simulink model "PDControllerModifiedToWork"  (R2020b)
settings: Solver=VariableStepAuto  StartTime=0.0  StopTime=30  RelTol=1e-3
values from neighbouring files (symbols this model uses):
  Arm = dhfunc(descriptor,d,a,alpha,theta,m,I,r,G,Jm,fv)    [Test.m]    (also in TestZone.m = dhfunc(descriptor,d,a,alpha,theta,m,I,r,G,Jm, Fv); TestZone2.m = dhfunc(descriptor,d,a,alpha,theta,m,I,r,G,Jm, Fc, Fv); TestZone2WithSingularity.m = dhfunc(descriptor,d,a,alpha,theta,m,I,r,G,Jm, Fv); dhfunc.m = SerialLink(LinkList, 'name', 'Arm'))
  Kd = eye(6)*kd    [TestZone.m]    (also in TestZone2.m = eye(3)*kd; TestZone2WithSingularity.m; Workspace.mat = [1 0 0 0 0 0 0 1 0 0 0 0 ... (36 elements, 6x6)])
  Kp = eye(6)*kp    [TestZone.m]    (also in TestZone2.m = eye(3)*kp; TestZone2WithSingularity.m; Workspace.mat = [1 0 0 0 0 0 0 1 0 0 0 0 ... (36 elements, 6x6)])
  Od = [1 0 0 1; 0 1 0 2; 0 0 1 3; 0 0 0 1]    [TestZone.m]    (also in Workspace.mat = [0.764842187284 0.644217687238 0 0 -0.644217687238 0.7648421)
  qdintial = [0,0,0,0,0,0]    [TestZone.m]    (also in Workspace.mat = [0 0 0])
  qintial = [0,0,0,0,0,0]    [TestZone.m]    (also in Workspace.mat = [0 0 0])
libraries: roblocks x1
settings Model: Creator=William Weiss  LastModifiedBy=kylej

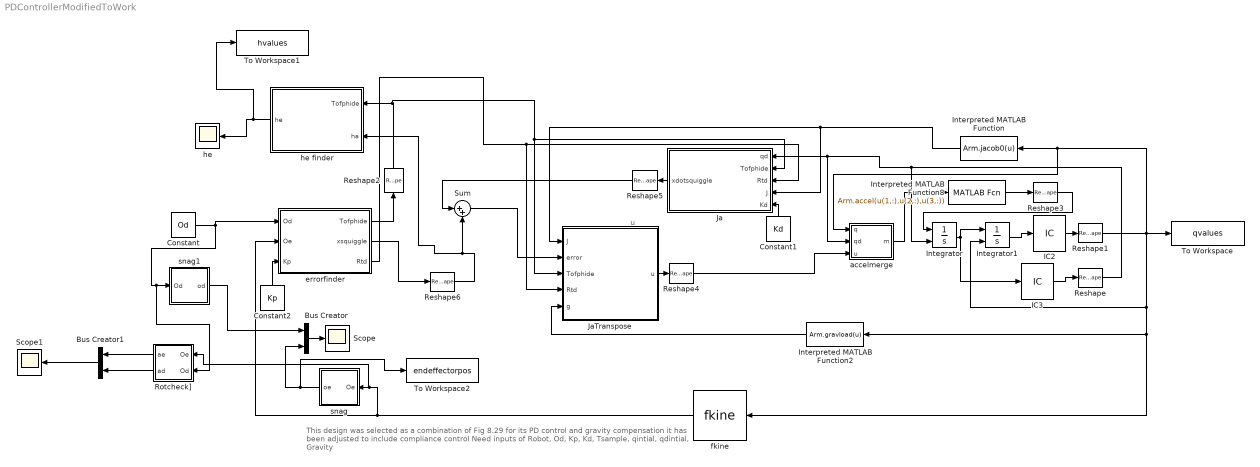
== system PDControllerModifiedToWork ==
  note: This design was selected as a combination of Fig 8.29 for its PD control and gravity compensation
      | it has been adjusted to include compliance control
      |
      | Need inputs of Robot, Od, Kp, Kd, Tsample, qintial, qdintial, Gravity
  note: u
  Bus Creator : BusCreator  Inputs=2
  Bus Creator1 : BusCreator  Inputs=2
  Constant : Constant  Value=Od
  Constant1 : Constant  Value=Kd
  Constant2 : Constant  Value=Kp
  IC2 : InitialCondition  Value=qintial
  IC3 : InitialCondition  Value=qdintial
  Integrator : Integrator  InitialConditionSource=external  ZeroCross=off
  Integrator1 : Integrator  InitialConditionSource=external  ZeroCross=off
  Interpreted MATLAB Function : MATLABFcn  MATLABFcn=Arm.jacob0(u)  Output1D=off
  Interpreted MATLAB Function2 : MATLABFcn  MATLABFcn=Arm.gravload(u)  Output1D=off
  Interpreted MATLAB Function8 : MATLABFcn  MATLABFcn=Arm.accel(u(1,:),u(2,:),u(3,:))  Output1D=off
  Ja : MATLAB Function  TreatAsAtomicUnit=on
  JaTranspose : MATLAB Function  TreatAsAtomicUnit=on
  Reshape{,1,3..6} (6 alike) : Reshape  OutputDimensionality=Row vector (2-D)
  Reshape2 : Reshape  OutputDimensionality=Customize  OutputDimensions=[3,3]
  Rotcheck] : MATLAB Function  TreatAsAtomicUnit=on
  Scope : Scope
  Scope1 : Scope
  Sum : Sum  Inputs=|++
  To Workspace : ToWorkspace  VariableName=qvalues  SaveFormat=Timeseries  SampleTime=-1
  To Workspace1 : ToWorkspace  VariableName=hvalues  SaveFormat=Timeseries  SampleTime=-1
  To Workspace2 : ToWorkspace  VariableName=endeffectorpos  SaveFormat=Timeseries  SampleTime=-1
  accelmerge : MATLAB Function  TreatAsAtomicUnit=on
  errorfinder : MATLAB Function  TreatAsAtomicUnit=on
  fkine : roblocks/Arm/fkine  robot=Arm
  he : Scope
  he finder : MATLAB Function  TreatAsAtomicUnit=on
  snag : MATLAB Function  TreatAsAtomicUnit=on
  snag1 : MATLAB Function  TreatAsAtomicUnit=on
  wires:
  Constant/1 -> Rotcheck]/2(Od), snag1/1(Od), errorfinder/1(Od)
  errorfinder/2(xsquiggle) -> Reshape6/1
  Ja/1(xdotsquiggle) -> Reshape5/1
  Sum/1 -> JaTranspose/2(error)
  errorfinder/3(Rtd) -> JaTranspose/4(Rtd), Ja/3(Rtd)
  he finder/1(he) -> To Workspace1/1, he/1
  Reshape/1 -> Integrator/2, accelmerge/2(qd), Ja/1(qd)
  Reshape1/1 -> To Workspace/1, accelmerge/1(q), Interpreted MATLAB Function/1, fkine/1, Interpreted MATLAB Function2/1, Integrator1/2
  Interpreted MATLAB Function/1 -> Ja/4(J), JaTranspose/1(J)
  Interpreted MATLAB Function8/1 -> Reshape3/1
  Reshape3/1 -> Integrator/1
  Integrator1/1 -> IC2/1
  Integrator/1 -> IC3/1, Integrator1/1
  IC3/1 -> Reshape/1
  IC2/1 -> Reshape1/1
  accelmerge/1(m) -> Interpreted MATLAB Function8/1
  JaTranspose/1(u) -> Reshape4/1
  errorfinder/1(Tofphide) -> Reshape2/1
  Reshape2/1 -> Ja/2(Tofphide), JaTranspose/3(Tofphide), he finder/1(Tofphide)
  snag/1(oe) -> To Workspace2/1, Bus Creator/2
  Bus Creator/1 -> Scope/1
  snag1/1(od) -> Bus Creator/1
  Constant1/1 -> Ja/5(Kd)
  Interpreted MATLAB Function2/1 -> JaTranspose/5(g)
  Constant2/1 -> errorfinder/3(Kp)
  Reshape4/1 -> accelmerge/3(u)
  Reshape5/1 -> Sum/1
  Reshape6/1 -> he finder/2(ha), Sum/2
  fkine/1 -> Rotcheck]/1(Oe), snag/1(Oe), errorfinder/2(Oe)
  Rotcheck]/2(ad) -> Bus Creator1/2
  Rotcheck]/1(ae) -> Bus Creator1/1
  Bus Creator1/1 -> Scope1/1

== matlab function PDControllerModifiedToWork/snag ==
  data: Oe input; oe output
function oe  = snag(Oe)
oe = Oe(1:3,4);
end

== matlab function PDControllerModifiedToWork/errorfinder ==
  data: Tofphide output; Od input; Oe input; xsquiggle output; Rtd output; Kp input
function [Tofphide,xsquiggle,Rtd] = errorfinder(Od,Oe,Kp)
%Od = 4x4 desired endvector postion and rotation
%Oe = 4x4 actual endvector postion and rotation
Te = Oe; %These are from the equation above 9.8 in the book just
Td = Od; %Just using these lines to maintain notation 

Rtd = Td(1:3,1:3).'; %Grabbing transpose of desired rotation for use later


Tde = inv(Td)*Te; %9.8 from the book

odde = Tde(1:3,4); %3x1 vector of the postions 
                  

Tofphide = Tde(1:3,1:3); %Snaging The rotation matrix for ease of use later


%issues with finding the euler angles of the transformation matrix.
phide = tform2eul(Tde,'XYZ'); %euler transformation using corke


xsquiggle = -[odde; phide'];
xsquiggle = Kp*xsquiggle;
end

== matlab function PDControllerModifiedToWork/JaTranspose ==
  data: J input; u output; error input; Tofphide input; Rtd input; g input
function u = Jatranspose(J,error,Tofphide,Rtd,g)
%Looking at eq 9.15 we must use Jad again


%Below is eq 9.14 to find JAd
Jad = inv([eye(3), zeros(3); zeros(3), Tofphide])*[Rtd, zeros(3); zeros(3), Rtd] *J;

%As described in 9.15 we must multiply Kpx-etc by Jtad
%error is kpxsquiggle - Kd Jad*qdot

%This below line should ensure that ones gravity is added 
%u is correct for the compliance method
u = g'+(Jad'*error');
end

== matlab function PDControllerModifiedToWork/accelmerge ==
  data: m output; q input; qd input; u input
function m = m(q, qd, u)
% he = inv(Tofphide)*ha;
m = [q;qd;u];
end

== matlab function PDControllerModifiedToWork/snag1 ==
  data: Od input; od output
function od  = snag(Od)
od = Od(1:3,4);
end

== matlab function PDControllerModifiedToWork/Ja ==
  data: xdotsquiggle output; qd input; Tofphide input; Rtd input; J input; Kd input
function xdotsquiggle = Ja(qd,Tofphide,Rtd,J,Kd)
%To validate the equation in 9.14 we need Tof phide
%Now that this is an input we can use it 

%J is just the jacobian of the robot at this q


%Below is from eq 9.14
Jad = inv([eye(3), zeros(3); zeros(3), Tofphide])*[Rtd, zeros(3); zeros(3), Rtd] *J;

%Now just finding xdotsquiggle from eq 9.13
xdotsquiggle = -Kd*Jad*qd';
end

== matlab function PDControllerModifiedToWork/he finder ==
  data: he output; Tofphide input; ha input
function he  = hefinder(Tofphide,ha)
he = inv([eye(3), zeros(3); zeros(3), Tofphide])*ha';
end

== matlab function PDControllerModifiedToWork/Rotcheck] ==
  data: Oe input; ae output; Od input; ad output
function [ae,ad]  = RotCheck(Oe,Od)
ae = tform2eul(Oe);
ad = tform2eul(Od);
end
